simulink model "power_13NodeTestFeeder_4VSC_PV_DEG_symmtrc_loads_"  (R2024b)
settings: Solver=ode15s  StartTime=0.0  StopTime=5  FixedStep=1e-6  MaxStep=1e-4  RelTol=1e-6  AbsTol=1e-8  EnableMultiTasking=on
PreLoadFcn:
  | %power_13NodeTestFeeder_init;
values from neighbouring files (symbols this model uses):
  a = 1.3    [init_para_with_symmtrc_loads.m]
  Cdc = 278e-3    (= 0.278)    [init_para_with_symmtrc_loads.m]
  fg = 60    [a01_scan_VSC_13_feeder.m]    (also in init_para_with_symmtrc_loads.m)
  Gn = 1000    [init_para_with_symmtrc_loads.m]
  H = 8    [init_para_with_symmtrc_loads.m]
  Ipv_n = Isc_n*(Rp+Rs)/Rp    (= 8.21426513558)    [init_para_with_symmtrc_loads.m]
  Isc_n = 8.21    [init_para_with_symmtrc_loads.m]
  k = 1.3806503e-23    [init_para_with_symmtrc_loads.m]    (also in ypm_plot_compare_ana_meas.m = 2)
  Kdroop = Sn/(Rdroop*60)    (= 4166666.66667)    [init_para_with_symmtrc_loads.m]
  KI = 0.0032    [init_para_with_symmtrc_loads.m]
  Ki_C = Rc/tau_C    (= 0.768)    [init_para_with_symmtrc_loads.m]
  Ki_DC = omega_DC^2*Cdc    [init_para_with_symmtrc_loads.m]
  ki_dvpp = kp_dvpp/Ti_dvpp    [init_para_with_symmtrc_loads.m]
  Ki_P = 1/(Ki_pq*tau_P)    [init_para_with_symmtrc_loads.m]
  Ki_PLL = Kp_PLL/tau_PLL    [init_para_with_symmtrc_loads.m]
  Kp_C = Lc/tau_C    (= 0.020372)    [init_para_with_symmtrc_loads.m]
  Kp_DC = 2*xi_DC*omega_DC*Cdc    [init_para_with_symmtrc_loads.m]
  kp_dvpp = -(2*Kdcgain)^-1    [init_para_with_symmtrc_loads.m]
  Kp_P = tau_C/(Ki_pq*tau_P)    [init_para_with_symmtrc_loads.m]
  Kp_PLL = xi_PLL*2*omega_PLL/Vp    [init_para_with_symmtrc_loads.m]
  KV = -0.123    [init_para_with_symmtrc_loads.m]
  kv_Vp = [ 1.021 1.042 1.0174]    [init_para_with_symmtrc_loads.m]
  KVmp = Vmp_n/Voc_n    (= 0.799392097264)    [init_para_with_symmtrc_loads.m]
  Lc = 20.372e-6    (= 2.0372e-05)    [init_para_with_symmtrc_loads.m]
  Lg = Xg /(2*pi*fg)    [init_para_with_symmtrc_loads.m]
  Np = 345    [init_para_with_symmtrc_loads.m]
  Ns = 45    [init_para_with_symmtrc_loads.m]
  Ns_cell = 54    [init_para_with_symmtrc_loads.m]
  p_jump_time = 5    [init_para_with_symmtrc_loads.m]
  p_jump_value = 2*-1e6    (= -2000000)    [init_para_with_symmtrc_loads.m]
  phi_vec = phi_vec_deg/180*pi    [init_para_with_symmtrc_loads.m]
  ppv_nom = 4.9687e+05    (= 496870)    [init_para_with_symmtrc_loads.m]
  q = 1.6021764e-19    [init_para_with_symmtrc_loads.m]
  Rc = 0.768e-3    (= 0.000768)    [init_para_with_symmtrc_loads.m]
  Rg = (U_rms^2 / S_sc) / (sqrt(1 + XoverR^2))    [init_para_with_symmtrc_loads.m]
  Rp = 425.405    [init_para_with_symmtrc_loads.m]
  Rs = 0.221    [init_para_with_symmtrc_loads.m]
  S_base_all = 1    [init_para_with_symmtrc_loads.m]
  Sn = 15e6    (= 15000000)    [init_para_with_symmtrc_loads.m]
  tau_PLL = 2*xi_PLL/omega_PLL    [init_para_with_symmtrc_loads.m]
  Tn = 25    [init_para_with_symmtrc_loads.m]
  Ts = T_ctrl/n_ctrl    [a01_scan_VSC_13_feeder.m]    (also in init_para_with_symmtrc_loads.m = 5e-05)
  U_rms = 4160    [init_para_with_symmtrc_loads.m]
  Vdc = 1200    [init_para_with_symmtrc_loads.m]
  Voc_n = 32.9    [init_para_with_symmtrc_loads.m]
  Vp = sqrt(2)*480/sqrt(3)    [a01_scan_VSC_13_feeder.m]    (also in init_para_with_symmtrc_loads.m = Ug*sqrt(2)/sqrt(3))
undefined symbols (not defined in the file or in its folder): j, Newton, para_grid, para_PVgeno, Raphson
libraries: spsabctoAlphaBetaZeroLib x141, spsPower3phInstantaneousLib x70, spsSeriesRLCBranchLib x44, spsThreePhaseVIMeasurementLib x27, slpidlib x24, spsThreePhaseSeriesRLCLoadLib x15, spsControlledVoltageSourceLib x15, spsMeanLib x9, spsCurrentMeasurementLib x8, spsControlledCurrentSourceLib x8, cstblocks x8, spsGroundLib x5
(part 1 of 10)
settings Model: Creator=MathWorks  LastModifiedBy=clubbert
settings DataIOCC: ExternalInput=getinputstruct(op_IEEE_13_node_5)  InitialState=getstatestruct(op_IEEE_13_node_5)  LimitDataPoints=on  SaveFormat=Array  SignalLoggingSaveFormat=ModelDataLogs  ReturnWorkspaceOutputs=off
settings OptimizationCC: ExpressionDepthLimit=2147483647  LifeSpan=inf
settings DebuggingCC: UnderspecifiedInitializationDetection=Classic  MergeDetectMultiDrivingBlocksExec=none  FcnCallInpInsideContextMsg=warning  AllowSymbolicDim=off  StateNameClashWarn=warning  SFUnexpectedBacktrackingDiag=warning  SFNoUnconditionalDefaultTransitionDiag=warning  SFExecutionAtInitializationDiag=none  ArithmeticOperatorsInVariantConditions=warning
settings HardwareCC: ProdBitPerPointer=32  ProdBitPerSizeT=32  ProdBitPerPtrDiffT=32  ProdLargestAtomicFloat=None  ProdIntDivRoundTo=Undefined  ProdEndianess=Unspecified  ProdWordSize=32  ProdHWDeviceType=32-bit Generic
settings ModelReferenceCC: EnableRefExpFcnMdlSchedulingChecks=on  PropagateSignalLabelsOutOfModel=off
settings SFSimCC: SimUseLocalCustomCode=off  CustomCodeUndefinedFunction=UseInterfaceOnly
settings RTWCC: RTWUseLocalCustomCode=off  GPUComputeCapability=3.5
settings CodeAppCC: StateflowObjectComments=on
settings GRTTargetCC: TargetLangStandard=C89/C90 (ANSI)  CombineOutputUpdateFcns=off  GRTInterface=on
settings ConfigComp: CovMetricSettings=dw  CovSaveCumulativeToWorkspaceVar=on  CovSaveSingleToWorkspaceVar=on  CovExternalEMLEnable=off  CovSFcnEnable=off
settings SimscapeCC: SimscapeNormalizeSystem=off

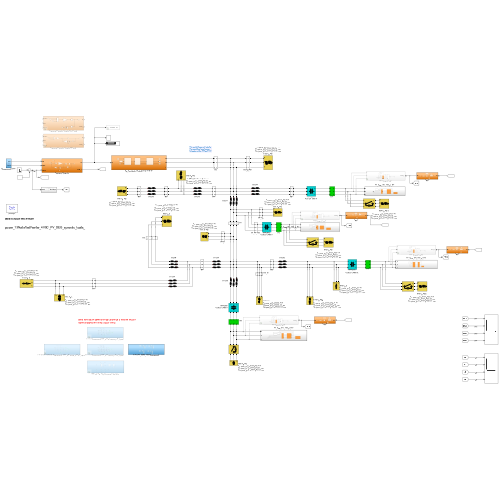
[thumbnail: Simulink's stored preview of the top-level diagram]
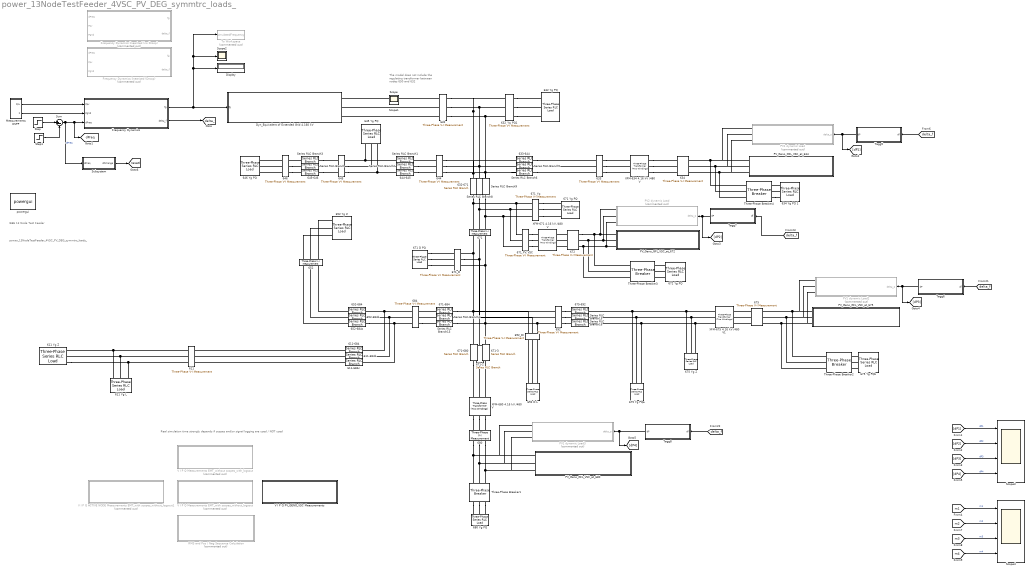
== system power_13NodeTestFeeder_4VSC_PV_DEG_symmtrc_loads_ ==
  note: Real simulation time strongly depends if scopes and/or
      | signal logging are used / NOT used
  note: power_13NodeTestFeeder_4VSC_PV_DEG_symmtrc_loads_
  note: IEEE 13 Node Test Feeder
  note: The model does not include
      | the regulating transformer
      | between nodes 650 and 632
  " 634 Yg PQ 1" : spsThreePhaseSeriesRLCLoadLib/Three-Phase Series RLC Load  LConnTagsString=A|B|C  Configuration=Y (grounded)  NominalVoltage=120e3  Vabc=para_grid.n634YgPQ.V_LN_rms  Vabcp=[1e3 1e3 1e3]  NominalFrequency=fg  UnbalancedPower=on  ActivePower=1e+006  InductivePower=0  CapacitivePower=0  Pabc=para_grid.n634YgPQ.P  QLabc=para_grid.n634YgPQ.QL  QCabc=para_grid.n634YgPQ.QC  Pabcp=[10e3 9e3 11e3]  QLabcp=[100 90 110]  QCabcp=[100 90 110]  Measurements=None  LoadType=constant PQ
      settings: AttributesFormatString=|
      | P= %<Pabc> W
      | Ql=%<QLabc> var
      | Qc=%<QCabc> var
  " 645 Yg PQ" : spsThreePhaseSeriesRLCLoadLib/Three-Phase Series RLC Load  LConnTagsString=A|B|C  Configuration=Y (grounded)  NominalVoltage=120e3  Vabc=para_grid.n645YgPQ.V_LN_rms  Vabcp=[1e3 1e3 1e3]  NominalFrequency=fg  UnbalancedPower=on  ActivePower=1e+006  InductivePower=0  CapacitivePower=0  Pabc=para_grid.n645YgPQ.P  QLabc=para_grid.n645YgPQ.QL  QCabc=para_grid.n645YgPQ.QC  Pabcp=[10e3 9e3 11e3]  QLabcp=[100 90 110]  QCabcp=[100 90 110]  Measurements=None  LoadType=constant PQ
      settings: AttributesFormatString=|
      | P= %<Pabc> W
      | Ql=%<QLabc> var
      | Qc=%<QCabc> var
  " 646 Yg PQ" : spsThreePhaseSeriesRLCLoadLib/Three-Phase Series RLC Load  LConnTagsString=A|B|C  Configuration=Y (grounded)  NominalVoltage=120e3  Vabc=para_grid.n646YgPQ.V_LN_rms  Vabcp=[1e3 1e3 1e3]  NominalFrequency=fg  UnbalancedPower=on  ActivePower=1e+006  InductivePower=0  CapacitivePower=0  Pabc=para_grid.n646YgPQ.P  QLabc=para_grid.n646YgPQ.QL  QCabc=para_grid.n646YgPQ.QC  Pabcp=[10e3 9e3 11e3]  QLabcp=[100 90 110]  QCabcp=[100 90 110]  Measurements=None  LoadType=constant PQ
      settings: AttributesFormatString=|
      | P= %<Pabc> W
      | Ql=%<QLabc> var
      | Qc=%<QCabc> var
  " 652 Yg Z" : spsThreePhaseSeriesRLCLoadLib/Three-Phase Series RLC Load  LConnTagsString=A|B|C  Configuration=Y (grounded)  NominalVoltage=120e3  Vabc=para_grid.n652YgZ.V_LN_rms  Vabcp=[1e3 1e3 1e3]  NominalFrequency=fg  UnbalancedPower=on  ActivePower=1e+006  InductivePower=0  CapacitivePower=0  Pabc=para_grid.n652YgZ.P  QLabc=para_grid.n652YgZ.QL  QCabc=para_grid.n652YgZ.QC  Pabcp=[10e3 9e3 11e3]  QLabcp=[100 90 110]  QCabcp=[100 90 110]  Measurements=None  LoadType=constant PQ
      settings: AttributesFormatString=|
      | P= %<Pabc> W
      | Ql=%<QLabc> var
      | Qc=%<QCabc> var
  " 672 Yg PQ " : spsThreePhaseSeriesRLCLoadLib/Three-Phase Series RLC Load  LConnTagsString=A|B|C  Configuration=Y (grounded)  NominalVoltage=120e3  Vabc=para_grid.n672YgPQ.V_LN_rms  Vabcp=[1e3 1e3 1e3]  NominalFrequency=fg  UnbalancedPower=on  ActivePower=1e+006  InductivePower=0  CapacitivePower=0  Pabc=para_grid.n672YgPQ.P  QLabc=para_grid.n672YgPQ.QL  QCabc=para_grid.n672YgPQ.QC  Pabcp=[10e3 9e3 11e3]  QLabcp=[100 90 110]  QCabcp=[100 90 110]  Measurements=None  LoadType=constant PQ
      settings: AttributesFormatString=|
      | P= %<Pabc> W
      | Ql=%<QLabc> var
      | Qc=%<QCabc> var
  " 675 Yg PQb " : spsThreePhaseSeriesRLCLoadLib/Three-Phase Series RLC Load  LConnTagsString=A|B|C  Configuration=Y (grounded)  NominalVoltage=120e3  Vabc=[ 0.993805 1.0218 0.995862]*277.128  Vabcp=[1e3 1e3 1e3]  NominalFrequency=60  UnbalancedPower=on  ActivePower=1e+006  InductivePower=0  CapacitivePower=0  Pabc=para_grid.n675YgPQb.P  QLabc=para_grid.n675YgPQb.QL  QCabc=para_grid.n675YgPQb.QC  Pabcp=[10e3 9e3 11e3]  QLabcp=[100 90 110]  QCabcp=[100 90 110]  Measurements=None  LoadType=constant PQ
      settings: AttributesFormatString=|
      | P= %<Pabc> W
      | Ql=%<QLabc> var
      | Qc=%<QCabc> var
  " 680 Yg PQ " : spsThreePhaseSeriesRLCLoadLib/Three-Phase Series RLC Load  LConnTagsString=A|B|C  Configuration=Y (grounded)  NominalVoltage=120e3  Vabc=para_grid.n680YgPQ.V_LN_rms  Vabcp=[1e3 1e3 1e3]  NominalFrequency=fg  UnbalancedPower=on  ActivePower=1e+006  InductivePower=0  CapacitivePower=0  Pabc=para_grid.n680YgPQ.P  QLabc=para_grid.n680YgPQ.QL  QCabc=para_grid.n680YgPQ.QC  Pabcp=[10e3 9e3 11e3]  QLabcp=[100 90 110]  QCabcp=[100 90 110]  Measurements=None  LoadType=constant PQ
      settings: AttributesFormatString=|
      | P= %<Pabc> W
      | Ql=%<QLabc> var
      | Qc=%<QCabc> var
  611 : spsThreePhaseVIMeasurementLib/Three-Phase V-I Measurement  VoltageMeasurement=phase-to-ground  SetLabelV=on  LabelV=Vabc_611  Vpu=off  VpuLL=off  CurrentMeasurement=yes  SetLabelI=on  LabelI=Iabc_611  Ipu=off  Pbase=100e6  Vbase=4160  OutputType=Complex  PhasorSimulation=off  PSBequivalent=0
  611 Yg L : spsThreePhaseSeriesRLCLoadLib/Three-Phase Series RLC Load  LConnTagsString=A|B|C  Configuration=Y (grounded)  NominalVoltage=120e3  Vabc=para_grid.n611YgL.V_LN_rms  Vabcp=para_grid.n671DPQ.V_LN_rms  NominalFrequency=fg  UnbalancedPower=on  ActivePower=1e+006  InductivePower=0  CapacitivePower=0  Pabc=para_grid.n611YgL.P  QLabc=para_grid.n611YgL.QL  QCabc=para_grid.n611YgL.QC  Pabcp=para_grid.n671DPQ.P  QLabcp=para_grid.n671DPQ.QL  QCabcp=para_grid.n671DPQ.QC  Measurements=None  LoadType=constant PQ
      settings: AttributesFormatString=|
      | P= %<Pabcp> W
      | Ql=%<QLabcp> var
      | Qc=%<QCabcp> var
  611 Yg Z : spsThreePhaseSeriesRLCLoadLib/Three-Phase Series RLC Load  LConnTagsString=A|B|C  Configuration=Y (grounded)  NominalVoltage=120e3  Vabc=para_grid.n611YgZ.V_LN_rms  Vabcp=para_grid.n671DPQ.V_LN_rms  NominalFrequency=fg  UnbalancedPower=on  ActivePower=1e+006  InductivePower=0  CapacitivePower=0  Pabc=para_grid.n611YgZ.P  QLabc=para_grid.n611YgZ.QL  QCabc=para_grid.n611YgZ.QC  Pabcp=para_grid.n671DPQ.P  QLabcp=para_grid.n671DPQ.QL  QCabcp=para_grid.n671DPQ.QC  Measurements=None  LoadType=constant PQ
      settings: AttributesFormatString=|
      | P= %<Pabcp> W
      | Ql=%<QLabcp> var
      | Qc=%<QCabcp> var
  611-684 : spsSeriesRLCBranchLib/Series RLC Branch  LConnTagsString=__new0  RConnTagsString=__new0  BranchType=RL  Resistance=para_grid.l611_684.R  Inductance=para_grid.l611_684.L  SetiL0=off  InitialCurrent=0  Capacitance=1e-6  Setx0=off  InitialVoltage=0  Measurements=None
  611-684b : spsSeriesRLCBranchLib/Series RLC Branch  LConnTagsString=__new0  RConnTagsString=__new0  BranchType=RL  Resistance=para_grid.l611_684.R  Inductance=para_grid.l611_684.L  SetiL0=off  InitialCurrent=0  Capacitance=1e-6  Setx0=off  InitialVoltage=0  Measurements=None
  611-684c : spsSeriesRLCBranchLib/Series RLC Branch  LConnTagsString=__new0  RConnTagsString=__new0  BranchType=RL  Resistance=para_grid.l611_684.R  Inductance=para_grid.l611_684.L  SetiL0=off  InitialCurrent=0  Capacitance=1e-6  Setx0=off  InitialVoltage=0  Measurements=None
  632 : spsThreePhaseVIMeasurementLib/Three-Phase V-I Measurement  VoltageMeasurement=phase-to-ground  SetLabelV=on  LabelV=Vabc_632  Vpu=off  VpuLL=off  CurrentMeasurement=yes  SetLabelI=on  LabelI=Iabc_632  Ipu=off  Pbase=100e6  Vbase=4160  OutputType=Complex  PhasorSimulation=off  PSBequivalent=0
  632 Yg PQ : spsThreePhaseSeriesRLCLoadLib/Three-Phase Series RLC Load  LConnTagsString=A|B|C  Configuration=Y (grounded)  NominalVoltage=120e3  Vabc=para_grid.n632YgPQ.V_LN_rms  Vabcp=[1e3 1e3 1e3]  NominalFrequency=fg  UnbalancedPower=on  ActivePower=1e+006  InductivePower=0  CapacitivePower=0  Pabc=para_grid.n632YgPQ.P  QLabc=para_grid.n632YgPQ.QL  QCabc=para_grid.n632YgPQ.QC  Pabcp=[10e3 9e3 11e3]  QLabcp=[100 90 110]  QCabcp=[100 90 110]  Measurements=None  LoadType=constant PQ
      settings: AttributesFormatString=|
      | P= %<Pabc> W
      | Ql=%<QLabc> var
      | Qc=%<QCabc> var
  632-671 : spsSeriesRLCBranchLib/Series RLC Branch  LConnTagsString=__new0  RConnTagsString=__new0  BranchType=RL  Resistance=para_grid.l632_671.R  Inductance=para_grid.l632_671.L  SetiL0=off  InitialCurrent=0  Capacitance=1e-6  Setx0=off  InitialVoltage=0  Measurements=None
  632_Yg_PQ1 : spsThreePhaseVIMeasurementLib/Three-Phase V-I Measurement  VoltageMeasurement=phase-to-ground  SetLabelV=on  LabelV=Vabc_632_Yg  Vpu=off  VpuLL=off  CurrentMeasurement=yes  SetLabelI=on  LabelI=Iabc_632_Yg  Ipu=off  Pbase=100e6  Vbase=4160  OutputType=Complex  PhasorSimulation=off  PSBequivalent=0
  633 : spsThreePhaseVIMeasurementLib/Three-Phase V-I Measurement  VoltageMeasurement=phase-to-ground  SetLabelV=on  LabelV=Vabc_633  Vpu=off  VpuLL=off  CurrentMeasurement=yes  SetLabelI=on  LabelI=Iabc_633  Ipu=off  Pbase=100e6  Vbase=4160  OutputType=Complex  PhasorSimulation=off  PSBequivalent=0
  633-644 : spsSeriesRLCBranchLib/Series RLC Branch  LConnTagsString=__new0  RConnTagsString=__new0  BranchType=RL  Resistance=para_grid.l633_644.R  Inductance=para_grid.l633_644.L  SetiL0=off  InitialCurrent=0  Capacitance=1e-6  Setx0=off  InitialVoltage=0  Measurements=None
  634 : spsThreePhaseVIMeasurementLib/Three-Phase V-I Measurement  VoltageMeasurement=phase-to-ground  SetLabelV=on  LabelV=Vabc_634  Vpu=off  VpuLL=off  CurrentMeasurement=yes  SetLabelI=on  LabelI=Iabc_634  Ipu=off  Pbase=100e6  Vbase=4160  OutputType=Complex  PhasorSimulation=off  PSBequivalent=0
  644 : spsThreePhaseVIMeasurementLib/Three-Phase V-I Measurement  VoltageMeasurement=phase-to-ground  SetLabelV=on  LabelV=Vabc_644  Vpu=off  VpuLL=off  CurrentMeasurement=yes  SetLabelI=on  LabelI=Iabc_644  Ipu=off  Pbase=100e6  Vbase=4160  OutputType=Complex  PhasorSimulation=off  PSBequivalent=0
  644-645 : spsSeriesRLCBranchLib/Series RLC Branch  LConnTagsString=__new0  RConnTagsString=__new0  BranchType=RL  Resistance=para_grid.l644_645.R  Inductance=para_grid.l644_645.L  SetiL0=off  InitialCurrent=0  Capacitance=1e-6  Setx0=off  InitialVoltage=0  Measurements=None
  645 : spsThreePhaseVIMeasurementLib/Three-Phase V-I Measurement  VoltageMeasurement=phase-to-ground  SetLabelV=on  LabelV=Vabc_645  Vpu=off  VpuLL=off  CurrentMeasurement=yes  SetLabelI=on  LabelI=Iabc_645  Ipu=off  Pbase=100e6  Vbase=4160  OutputType=Complex  PhasorSimulation=off  PSBequivalent=0
  645-646 : spsSeriesRLCBranchLib/Series RLC Branch  LConnTagsString=__new0  RConnTagsString=__new0  BranchType=RL  Resistance=para_grid.l645_646.R  Inductance=para_grid.l645_646.L  SetiL0=off  InitialCurrent=0  Capacitance=1e-6  Setx0=off  InitialVoltage=0  Measurements=None
  646 : spsThreePhaseVIMeasurementLib/Three-Phase V-I Measurement  VoltageMeasurement=phase-to-ground  SetLabelV=on  LabelV=Vabc_646  Vpu=off  VpuLL=off  CurrentMeasurement=yes  SetLabelI=on  LabelI=Iabc_646  Ipu=off  Pbase=100e6  Vbase=4160  OutputType=Complex  PhasorSimulation=off  PSBequivalent=0
  652 : spsThreePhaseVIMeasurementLib/Three-Phase V-I Measurement  VoltageMeasurement=phase-to-ground  SetLabelV=on  LabelV=Vabc_652  Vpu=off  VpuLL=off  CurrentMeasurement=yes  SetLabelI=on  LabelI=Iabc_652  Ipu=off  Pbase=100e6  Vbase=4160  OutputType=Complex  PhasorSimulation=off  PSBequivalent=0
  652-684 : spsSeriesRLCBranchLib/Series RLC Branch  LConnTagsString=__new0  RConnTagsString=__new0  BranchType=RL  Resistance=para_grid.l652_684.R  Inductance=para_grid.l652_684.L  SetiL0=off  InitialCurrent=0  Capacitance=1e-6  Setx0=off  InitialVoltage=0  Measurements=None
  652-684b : spsSeriesRLCBranchLib/Series RLC Branch  LConnTagsString=__new0  RConnTagsString=__new0  BranchType=RL  Resistance=para_grid.l652_684.R  Inductance=para_grid.l652_684.L  SetiL0=off  InitialCurrent=0  Capacitance=1e-6  Setx0=off  InitialVoltage=0  Measurements=None
  652-684c : spsSeriesRLCBranchLib/Series RLC Branch  LConnTagsString=__new0  RConnTagsString=__new0  BranchType=RL  Resistance=para_grid.l652_684.R  Inductance=para_grid.l652_684.L  SetiL0=off  InitialCurrent=0  Capacitance=1e-6  Setx0=off  InitialVoltage=0  Measurements=None
  671 : spsThreePhaseVIMeasurementLib/Three-Phase V-I Measurement  VoltageMeasurement=phase-to-ground  SetLabelV=on  LabelV=Vabc_671  Vpu=off  VpuLL=off  CurrentMeasurement=yes  SetLabelI=on  LabelI=Iabc_671  Ipu=off  Pbase=100e6  Vbase=4160  OutputType=Complex  PhasorSimulation=off  PSBequivalent=0
  671 D PQ : spsThreePhaseSeriesRLCLoadLib/Three-Phase Series RLC Load  LConnTagsString=A|B|C  Configuration=Delta  NominalVoltage=120e3  Vabc="[1  1  1]*120e3/sqrt(3)"  Vabcp=para_grid.n671DPQ.V_LN_rms  NominalFrequency=fg  UnbalancedPower=on  ActivePower=1e+006  InductivePower=0  CapacitivePower=0  Pabc="[17 66  117]*1e3/2"  QLabc="[10 38  68]*1e3/2"  QCabc=[0 0 0]  Pabcp=para_grid.n671DPQ.P  QLabcp=para_grid.n671DPQ.QL  QCabcp=para_grid.n671DPQ.QC  Measurements=None  LoadType=constant PQ
      settings: AttributesFormatString=|
      | P= %<Pabcp> W
      | Ql=%<QLabcp> var
      | Qc=%<QCabcp> var
  671 Yg PQ : spsThreePhaseSeriesRLCLoadLib/Three-Phase Series RLC Load  LConnTagsString=A|B|C  Configuration=Y (grounded)  NominalVoltage=120e3  Vabc=para_grid.n671YgPQ.V_LN_rms  Vabcp=[1e3 1e3 1e3]  NominalFrequency=fg  UnbalancedPower=on  ActivePower=1e+006  InductivePower=0  CapacitivePower=0  Pabc=para_grid.n671YgPQ.P  QLabc=para_grid.n671YgPQ.QL  QCabc=para_grid.n671YgPQ.QC  Pabcp=[10e3 9e3 11e3]  QLabcp=[100 90 110]  QCabcp=[100 90 110]  Measurements=None  LoadType=constant PQ
      settings: AttributesFormatString=|
      | P= %<Pabc> W
      | Ql=%<QLabc> var
      | Qc=%<QCabc> var
  671-2 : spsSeriesRLCBranchLib/Series RLC Branch  LConnTagsString=__new0  RConnTagsString=__new0  BranchType=RL  Resistance=para_grid.l671_680.R  Inductance=para_grid.l671_680.L  SetiL0=off  InitialCurrent=0  Capacitance=1e-6  Setx0=off  InitialVoltage=0  Measurements=None
  671-3 : spsSeriesRLCBranchLib/Series RLC Branch  LConnTagsString=__new0  RConnTagsString=__new0  BranchType=RL  Resistance=para_grid.l671_680.R  Inductance=para_grid.l671_680.L  SetiL0=off  InitialCurrent=0  Capacitance=1e-6  Setx0=off  InitialVoltage=0  Measurements=None
  671-680 : spsSeriesRLCBranchLib/Series RLC Branch  LConnTagsString=__new0  RConnTagsString=__new0  BranchType=RL  Resistance=para_grid.l671_680.R  Inductance=para_grid.l671_680.L  SetiL0=off  InitialCurrent=0  Capacitance=1e-6  Setx0=off  InitialVoltage=0  Measurements=None
  671-684 : spsSeriesRLCBranchLib/Series RLC Branch  LConnTagsString=__new0  RConnTagsString=__new0  BranchType=RL  Resistance=para_grid.l671_684.R  Inductance=para_grid.l671_684.L  SetiL0=off  InitialCurrent=0  Capacitance=1e-6  Setx0=off  InitialVoltage=0  Measurements=None
  671_D : spsThreePhaseVIMeasurementLib/Three-Phase V-I Measurement  VoltageMeasurement=phase-to-ground  SetLabelV=on  LabelV=Vabc_671_D  Vpu=off  VpuLL=off  CurrentMeasurement=yes  SetLabelI=on  LabelI=Iabc_671_D  Ipu=off  Pbase=100e6  Vbase=4160  OutputType=Complex  PhasorSimulation=off  PSBequivalent=0
  671_PV_VSC : spsThreePhaseVIMeasurementLib/Three-Phase V-I Measurement  VoltageMeasurement=phase-to-ground  SetLabelV=on  LabelV=Vabc_671_VSC  Vpu=off  VpuLL=off  CurrentMeasurement=yes  SetLabelI=on  LabelI=Iabc_671_VSC  Ipu=off  Pbase=100e6  Vbase=4160  OutputType=Complex  PhasorSimulation=off  PSBequivalent=0
  671_Yg : spsThreePhaseVIMeasurementLib/Three-Phase V-I Measurement  VoltageMeasurement=phase-to-ground  SetLabelV=on  LabelV=Vabc_671_Yg  Vpu=off  VpuLL=off  CurrentMeasurement=yes  SetLabelI=on  LabelI=Iabc_671_Yg  Ipu=off  Pbase=100e6  Vbase=4160  OutputType=Complex  PhasorSimulation=off  PSBequivalent=0
  672 : spsThreePhaseVIMeasurementLib/Three-Phase V-I Measurement  VoltageMeasurement=phase-to-ground  SetLabelV=on  LabelV=Vabc_672  Vpu=off  VpuLL=off  CurrentMeasurement=yes  SetLabelI=on  LabelI=Iabc_672  Ipu=off  Pbase=100e6  Vbase=4160  OutputType=Complex  PhasorSimulation=off  PSBequivalent=0
  675 : spsThreePhaseVIMeasurementLib/Three-Phase V-I Measurement  VoltageMeasurement=phase-to-ground  SetLabelV=on  LabelV=Vabc_675  Vpu=off  VpuLL=off  CurrentMeasurement=yes  SetLabelI=on  LabelI=Iabc_675  Ipu=off  Pbase=100e6  Vbase=4160  OutputType=Complex  PhasorSimulation=off  PSBequivalent=0
  675 Yg PQa : spsThreePhaseSeriesRLCLoadLib/Three-Phase Series RLC Load  LConnTagsString=A|B|C  Configuration=Y (grounded)  NominalVoltage=120e3  Vabc=para_grid.n675YgPQa.V_LN_rms  Vabcp=[1e3 1e3 1e3]  NominalFrequency=fg  UnbalancedPower=on  ActivePower=1e+006  InductivePower=0  CapacitivePower=0  Pabc=para_grid.n675YgPQa.P  QLabc=para_grid.n675YgPQa.QL  QCabc=para_grid.n675YgPQa.QC  Pabcp=[10e3 9e3 11e3]  QLabcp=[100 90 110]  QCabcp=[100 90 110]  Measurements=None  LoadType=constant PQ
      settings: AttributesFormatString=|
      | P= %<Pabc> W
      | Ql=%<QLabc> var
      | Qc=%<QCabc> var
  675 Yg Z : spsThreePhaseSeriesRLCLoadLib/Three-Phase Series RLC Load  LConnTagsString=A|B|C  Configuration=Y (grounded)  NominalVoltage=120e3  Vabc=para_grid.n675YgZ.V_LN_rms  Vabcp=[1e3 1e3 1e3]  NominalFrequency=fg  UnbalancedPower=on  ActivePower=1e+006  InductivePower=0  CapacitivePower=0  Pabc=para_grid.n675YgZ.P  QLabc=para_grid.n675YgZ.QL  QCabc=para_grid.n675YgZ.QC  Pabcp=[10e3 9e3 11e3]  QLabcp=[100 90 110]  QCabcp=[100 90 110]  Measurements=None  LoadType=constant Z
      settings: AttributesFormatString=|
      | P= %<Pabc> W
      | Ql=%<QLabc> var
      | Qc=%<QCabc> var
  675-692 : spsSeriesRLCBranchLib/Series RLC Branch  LConnTagsString=__new0  RConnTagsString=__new0  BranchType=RL  Resistance=para_grid.l675_692.R  Inductance=para_grid.l675_692.L  SetiL0=off  InitialCurrent=0  Capacitance=1e-6  Setx0=off  InitialVoltage=0  Measurements=None
  680 : spsThreePhaseVIMeasurementLib/Three-Phase V-I Measurement  VoltageMeasurement=phase-to-ground  SetLabelV=on  LabelV=Vabc_680  Vpu=off  VpuLL=off  CurrentMeasurement=yes  SetLabelI=on  LabelI=Iabc_680  Ipu=off  Pbase=100e6  Vbase=4160  OutputType=Complex  PhasorSimulation=off  PSBequivalent=0
  684 : spsThreePhaseVIMeasurementLib/Three-Phase V-I Measurement  VoltageMeasurement=phase-to-ground  SetLabelV=on  LabelV=Vabc_684  Vpu=off  VpuLL=off  CurrentMeasurement=yes  SetLabelI=on  LabelI=Iabc_684  Ipu=off  Pbase=100e6  Vbase=4160  OutputType=Complex  PhasorSimulation=off  PSBequivalent=0
  692 : spsThreePhaseVIMeasurementLib/Three-Phase V-I Measurement  VoltageMeasurement=phase-to-ground  SetLabelV=on  LabelV=Vabc_692  Vpu=off  VpuLL=off  CurrentMeasurement=yes  SetLabelI=on  LabelI=Iabc_692  Ipu=off  Pbase=100e6  Vbase=4160  OutputType=Complex  PhasorSimulation=off  PSBequivalent=0
  692 D L : spsThreePhaseSeriesRLCLoadLib/Three-Phase Series RLC Load  LConnTagsString=A|B|C  Configuration=Delta  NominalVoltage=120e3  Vabc="[1  1  1]*120e3/sqrt(3)"  Vabcp=para_grid.n692DL.V_LN_rms  NominalFrequency=fg  UnbalancedPower=on  ActivePower=1e+006  InductivePower=0  CapacitivePower=0  Pabc="[17 66  117]*1e3/2"  QLabc="[10 38  68]*1e3/2"  QCabc=[0 0 0]  Pabcp=para_grid.n692DL.P  QLabcp=para_grid.n692DL.QL  QCabcp=para_grid.n692DL.QC  Measurements=None  LoadType=constant I
      settings: AttributesFormatString=|
      | P= %<Pabcp> W
      | Ql=%<QLabcp> var
      | Qc=%<QCabcp> var
  692_DI : spsThreePhaseVIMeasurementLib/Three-Phase V-I Measurement  VoltageMeasurement=phase-to-ground  SetLabelV=on  LabelV=Vabc_692_DI  Vpu=off  VpuLL=off  CurrentMeasurement=yes  SetLabelI=on  LabelI=Iabc_692_DI  Ipu=off  Pbase=100e6  Vbase=4160  OutputType=Complex  PhasorSimulation=off  PSBequivalent=0
  Display : Display
  Dyn_Equivalent of Extended Grid 4.160 kV : Subsystem
  Frequency Dynamics : Subsystem
  Frequency Dynamics linearized (Droop) : Subsystem  Commented=on
  Frequency Dynamics linearized (no Droop) : Subsystem  Commented=on
  Measurements DVPP : Subsystem
  PV1 dynamic Load : Subsystem  Commented=on
  PV1 dynamic Load2 : Subsystem  Commented=on
  PV1 dynamic Load3 : Subsystem  Commented=on
  PV2 dynamic Load : Subsystem  Commented=on
  PV_Geno_GFL_VSC_at_634 : Subsystem
  PV_Geno_GFL_VSC_at_672 : Subsystem
  PV_Geno_GFL_VSC_at_675 : Subsystem
  PV_Geno_GFL_VSC_at_680 : Subsystem
  "RMS and Pos / Neg Sequence Calculation " : Subsystem  Commented=on
  Scope2 : Scope
  Scope3 : Scope  NumInputPorts=4
  Scope4 : Scope  NumInputPorts=4
  Series RLC Branch : spsSeriesRLCBranchLib/Series RLC Branch  LConnTagsString=__new0  RConnTagsString=__new0  BranchType=RL  Resistance=para_grid.l645_646.R  Inductance=para_grid.l645_646.L  SetiL0=off  InitialCurrent=0  Capacitance=1e-6  Setx0=off  InitialVoltage=0  Measurements=None
  Series RLC Branch1 : spsSeriesRLCBranchLib/Series RLC Branch  LConnTagsString=__new0  RConnTagsString=__new0  BranchType=RL  Resistance=para_grid.l644_645.R  Inductance=para_grid.l644_645.L  SetiL0=off  InitialCurrent=0  Capacitance=1e-6  Setx0=off  InitialVoltage=0  Measurements=None
  Series RLC Branch13 : spsSeriesRLCBranchLib/Series RLC Branch  LConnTagsString=__new0  RConnTagsString=__new0  BranchType=RL  Resistance=para_grid.l671_684.R  Inductance=para_grid.l671_684.L  SetiL0=off  InitialCurrent=0  Capacitance=1e-6  Setx0=off  InitialVoltage=0  Measurements=None
  Series RLC Branch15 : spsSeriesRLCBranchLib/Series RLC Branch  LConnTagsString=__new0  RConnTagsString=__new0  BranchType=RL  Resistance=para_grid.l675_692.R  Inductance=para_grid.l675_692.L  SetiL0=off  InitialCurrent=0  Capacitance=1e-6  Setx0=off  InitialVoltage=0  Measurements=None
  Series RLC Branch16 : spsSeriesRLCBranchLib/Series RLC Branch  LConnTagsString=__new0  RConnTagsString=__new0  BranchType=RL  Resistance=para_grid.l675_692.R  Inductance=para_grid.l675_692.L  SetiL0=off  InitialCurrent=0  Capacitance=1e-6  Setx0=off  InitialVoltage=0  Measurements=None
  Series RLC Branch2 : spsSeriesRLCBranchLib/Series RLC Branch  LConnTagsString=__new0  RConnTagsString=__new0  BranchType=RL  Resistance=para_grid.l644_645.R  Inductance=para_grid.l644_645.L  SetiL0=off  InitialCurrent=0  Capacitance=1e-6  Setx0=off  InitialVoltage=0  Measurements=None
  Series RLC Branch3 : spsSeriesRLCBranchLib/Series RLC Branch  LConnTagsString=__new0  RConnTagsString=__new0  BranchType=RL  Resistance=para_grid.l645_646.R  Inductance=para_grid.l645_646.L  SetiL0=off  InitialCurrent=0  Capacitance=1e-6  Setx0=off  InitialVoltage=0  Measurements=None
  Series RLC Branch4 : spsSeriesRLCBranchLib/Series RLC Branch  LConnTagsString=__new0  RConnTagsString=__new0  BranchType=RL  Resistance=para_grid.l671_684.R  Inductance=para_grid.l671_684.L  SetiL0=off  InitialCurrent=0  Capacitance=1e-6  Setx0=off  InitialVoltage=0  Measurements=None
  Series RLC Branch5 : spsSeriesRLCBranchLib/Series RLC Branch  LConnTagsString=__new0  RConnTagsString=__new0  BranchType=RL  Resistance=para_grid.l633_644.R  Inductance=para_grid.l633_644.L  SetiL0=off  InitialCurrent=0  Capacitance=1e-6  Setx0=off  InitialVoltage=0  Measurements=None
  Series RLC Branch6 : spsSeriesRLCBranchLib/Series RLC Branch  LConnTagsString=__new0  RConnTagsString=__new0  BranchType=RL  Resistance=para_grid.l633_644.R  Inductance=para_grid.l633_644.L  SetiL0=off  InitialCurrent=0  Capacitance=1e-6  Setx0=off  InitialVoltage=0  Measurements=None
  Series RLC Branch8 : spsSeriesRLCBranchLib/Series RLC Branch  LConnTagsString=__new0  RConnTagsString=__new0  BranchType=RL  Resistance=para_grid.l632_671.R  Inductance=para_grid.l632_671.L  SetiL0=off  InitialCurrent=0  Capacitance=1e-6  Setx0=off  InitialVoltage=0  Measurements=None
  Series RLC Branch9 : spsSeriesRLCBranchLib/Series RLC Branch  LConnTagsString=__new0  RConnTagsString=__new0  BranchType=RL  Resistance=para_grid.l632_671.R  Inductance=para_grid.l632_671.L  SetiL0=off  InitialCurrent=0  Capacitance=1e-6  Setx0=off  InitialVoltage=0  Measurements=None
  Step : Step  Time=p_jump_time  After=p_jump_value  SampleTime=0
  Step1 : Step  Time=p_jump_time+10  After=p_jump_value  SampleTime=0
  Subsystem : Subsystem
  Sum : Sum  Inputs=|+-
  Tagg5 : Subsystem
  Tagg6 : Subsystem
  Tagg7 : Subsystem
  Tagg8 : Subsystem
  Three-Phase Breaker1 : spsThreePhaseBreakerLib/Three-Phase Breaker  InitialState=open  SwitchA=on  SwitchB=on  SwitchC=on  SwitchTimes=para_grid.n680YgPQ.ts  External=off  BreakerResistance=0.01  SnubberResistance=1e6  SnubberCapacitance=inf  Measurements=None
  Three-Phase Breaker2 : spsThreePhaseBreakerLib/Three-Phase Breaker  InitialState=open  SwitchA=on  SwitchB=on  SwitchC=on  SwitchTimes=para_grid.n675YgPQ.ts  External=off  BreakerResistance=0.01  SnubberResistance=1e6  SnubberCapacitance=inf  Measurements=None
  Three-Phase Breaker3 : spsThreePhaseBreakerLib/Three-Phase Breaker  InitialState=open  SwitchA=on  SwitchB=on  SwitchC=on  SwitchTimes=para_grid.n672YgPQ.ts  External=off  BreakerResistance=0.01  SnubberResistance=1e6  SnubberCapacitance=inf  Measurements=None
  Three-Phase Breaker4 : spsThreePhaseBreakerLib/Three-Phase Breaker  InitialState=open  SwitchA=on  SwitchB=on  SwitchC=on  SwitchTimes=para_grid.n634YgPQ.ts  External=off  BreakerResistance=0.01  SnubberResistance=1e6  SnubberCapacitance=inf  Measurements=None
  To Workspace : ToWorkspace  Commented=on  VariableName=simulatedFrequency  SaveFormat=Timeseries  SampleTime=Ts
  V I P Q ACTIVE NODE Measurements EMT_with scopes_without_logsout1 : Subsystem  Commented=on
  V I P Q Measurements EMT_with scopes_without_logsout : Subsystem  Commented=on
  V I P Q Measurements EMT_without scopes_with_logsout : Subsystem  Commented=on
  V I P Q PV_GENO_VSC Measurements : Subsystem
  XFM-634 4.16 kV /480 V : spsThreePhaseTransformerTwoWindingsLib/Three-Phase Transformer (Two Windings)  Winding1Connection=Yg  Winding2Connection=Yg  CoreType=Three single-phase transformers  SetSaturation=off  Hysteresis=off  DataFile='hysteresis'  SetInitialFlux=off  Measurements=None  UNITS=pu  NominalPower=[ 500e3 , 60 ]  Winding1=[4160 0.011 0.02]  Winding2=[480 0 0]  Rm=500  Lm=500  L0=0.5  Saturation=[0 0;0.0024 1.2;1 1.52]  InitialFluxes=[0.8 -0.8 0.7]  BreakLoop=off  DiscreteSolver=Trapezoidal iterative  DataType=off  TransfoNumber=1
  XFM-671 4.16 kV /480 V : spsThreePhaseTransformerTwoWindingsLib/Three-Phase Transformer (Two Windings)  Winding1Connection=Yg  Winding2Connection=Yg  CoreType=Three single-phase transformers  SetSaturation=off  Hysteresis=off  DataFile='hysteresis'  SetInitialFlux=off  Measurements=None  UNITS=pu  NominalPower=[ 500e3 , 60 ]  Winding1=[4160 0.011 0.02]  Winding2=[480 0 0]  Rm=500  Lm=500  L0=0.5  Saturation=[0 0;0.0024 1.2;1 1.52]  InitialFluxes=[0.8 -0.8 0.7]  BreakLoop=off  DiscreteSolver=Trapezoidal iterative  DataType=off  TransfoNumber=1
  XFM-675 4.16 kV /480 V1 : spsThreePhaseTransformerTwoWindingsLib/Three-Phase Transformer (Two Windings)  Winding1Connection=Yg  Winding2Connection=Yg  CoreType=Three single-phase transformers  SetSaturation=off  Hysteresis=off  DataFile='hysteresis'  SetInitialFlux=off  Measurements=None  UNITS=pu  NominalPower=[ 500e3 , 60 ]  Winding1=[4160 0.011 0.02]  Winding2=[480 0 0]  Rm=500  Lm=500  L0=0.5  Saturation=[0 0;0.0024 1.2;1 1.52]  InitialFluxes=[0.8 -0.8 0.7]  BreakLoop=off  DiscreteSolver=Trapezoidal iterative  DataType=off  TransfoNumber=1
  XFM-680 4.16 kV /480 V : spsThreePhaseTransformerTwoWindingsLib/Three-Phase Transformer (Two Windings)  Winding1Connection=Yg  Winding2Connection=Yg  CoreType=Three single-phase transformers  SetSaturation=off  Hysteresis=off  DataFile='hysteresis'  SetInitialFlux=off  Measurements=None  UNITS=pu  NominalPower=[ 500e3 , 60 ]  Winding1=[4160 0.011 0.02]  Winding2=[480 0 0]  Rm=500  Lm=500  L0=0.5  Saturation=[0 0;0.0024 1.2;1 1.52]  InitialFluxes=[0.8 -0.8 0.7]  BreakLoop=off  DiscreteSolver=Trapezoidal iterative  DataType=off  TransfoNumber=1
  powergui : spspowerguiLib/powergui  Priority=1  SimulationMode=Discrete  SampleTime=Ts  frequency=60  Iterations=50  frequencyindice=0  Pbase=100e3  ErrMax=0.0001  UnitsV=kV  UnitsW=kW  buscounter=0  FunctionMessages=off  echomessages=off  EnableUseOfTLC=off  CurrentSourceSwitches=off  DisableSnubberDevices=off  DisableRonSwitches=off  DisableVfSwitches=off  DisplayEquations=off  AutomaticDiscreteSolvers=off  SolverType=Tustin/Backward Euler (TBE)  Interpol=off  ExternalGateDelay=off  methode=off  Ts=0  x0status=blocks  SPID=off  SwTol=0  HookPort=off  NonlinearTolerance=1e-4  nMaxIteration=100  ContinueOnMaxIteration=off  RestoreLinks=warning  ResistiveCurrentMeasurement=off  Frange=[0:2:500]  Ylog=off  Xlog=on  ShowGrid=off  save=off  variable=ZData  structure=0  ZoomFFT=on  StartTime=0.0  cycles=1  DisplayStyle=1  fundamental=60  FreqAxis=off  MaxFrequency=1000  frequencyindicesteady=1  RmsSteady=1  display=off
  Scope : Scope
  Scope1 : Scope
  tag scope: dPreq=global, delta_f=global, resetI=global
  wires:
  Frequency Dynamics/2(delta_f) -> [delta_f]
  Frequency Dynamics/1(fg) -> Display/1, To Workspace/1, Scope2/1, Dyn_Equivalent of Extended Grid 4.160 kV/1(fg)
  Step/1 -> Sum/1
  Step1/1 -> Sum/2
  Measurements DVPP/2(Pgrid) -> Frequency Dynamics/2(Pgrid)
  Measurements DVPP/1(Ppv) -> Frequency Dynamics/1(Ppv)
  Sum/1 -> Subsystem/1(dPreq), [dPreq], Frequency Dynamics/3(dPreq)  "dPreq"
  [dP1] -> Scope3/1  "dP1"
  [dP2] -> Scope3/2  "dP2"
  [dP3] -> Scope3/3  "dP3"
  [dP4] -> Scope3/4  "dP4"
  Tagg5/1(dP) -> PV1 dynamic Load/1(delta_p), [dP1]
  Tagg7/1(dP) -> [dP2], PV2 dynamic Load/1(delta_p)
  Tagg6/1(dP) -> [dP3], PV1 dynamic Load2/1(delta_p)
  [delta_f] -> Tagg5/1(df)
  [delta_f] -> Tagg6/1(df)
  [delta_f] -> Tagg7/1(df)
  Tagg8/1(dP) -> [dP4], PV1 dynamic Load3/1(delta_p)
  [delta_f] -> Tagg8/1(df)
  Subsystem/1(dPchange) -> [resetI]
  [m4] -> Scope4/4  "m4"
  [m2] -> Scope4/2  "m2"
  [m1] -> Scope4/1  "m1"
  [m3] -> Scope4/3  "m3"
  connections:
  Series RLC Branch6/LConn1 -- Series RLC Branch9/LConn1 -- 644/LConn3 -- 632_Yg_PQ1/LConn3 -- 632/RConn3
  675 Yg PQa/LConn2 -- Series RLC Branch15/RConn1 -- 675 Yg Z/LConn2 -- XFM-675 4.16 kV /480 V1/LConn2
  675 Yg PQa/LConn3 -- Series RLC Branch16/RConn1 -- 675 Yg Z/LConn3 -- XFM-675 4.16 kV /480 V1/LConn3
  675 Yg PQa/LConn1 -- 675 Yg Z/LConn1 -- XFM-675 4.16 kV /480 V1/LConn1 -- 675-692/RConn1
  645/LConn2 -- Series RLC Branch2/LConn1 -- " 645 Yg PQ"/LConn2
  671-680/LConn1 -- 671-684/RConn1 -- 692/RConn1 -- 692_DI/LConn1 -- 671_D/LConn1 -- 671/RConn1
  611 Yg Z/LConn3 -- 611/RConn3 -- 611 Yg L/LConn3
  671_D/LConn2 -- 692_DI/LConn2 -- 692/RConn2 -- 671-2/LConn1 -- Series RLC Branch4/RConn1 -- 671/RConn2
  Series RLC Branch9/RConn1 -- 671/LConn3 -- 671_PV_VSC/RConn3 -- 671_Yg/RConn3
  632-671/LConn1 -- 632_Yg_PQ1/LConn1 -- 632/RConn1 -- 644/LConn1 -- 633-644/LConn1
  Series RLC Branch8/LConn1 -- 644/LConn2 -- Series RLC Branch5/LConn1 -- 632_Yg_PQ1/LConn2 -- 632/RConn2
  671 D PQ/LConn1 -- 671_D/RConn1
  671 D PQ/LConn2 -- 671_D/RConn2
  671 D PQ/LConn3 -- 671_D/RConn3
  671_Yg/LConn1 -- 671 Yg PQ/LConn1
  671_Yg/LConn2 -- 671 Yg PQ/LConn2
  671_Yg/LConn3 -- 671 Yg PQ/LConn3
  692 D L/LConn1 -- 692_DI/RConn1
  692 D L/LConn2 -- 692_DI/RConn2
  692 D L/LConn3 -- 692_DI/RConn3
  645/LConn3 -- 644-645/LConn1 -- " 645 Yg PQ"/LConn3
  Series RLC Branch/RConn1 -- 645/RConn2
  645-646/RConn1 -- 645/RConn3
  Series RLC Branch1/LConn1 -- 645/LConn1 -- " 645 Yg PQ"/LConn1
  Series RLC Branch3/LConn1 -- 646/LConn1
  646/RConn1 -- " 646 Yg PQ"/LConn1
  646/LConn2 -- Series RLC Branch/LConn1
  646/LConn3 -- 645-646/LConn1
  633-644/RConn1 -- 633/RConn1
  Series RLC Branch5/RConn1 -- 633/RConn2
  Series RLC Branch6/RConn1 -- 633/RConn3
  633/LConn1 -- XFM-634 4.16 kV /480 V/LConn1
  633/LConn2 -- XFM-634 4.16 kV /480 V/LConn2
  633/LConn3 -- XFM-634 4.16 kV /480 V/LConn3
  692_DI/LConn3 -- 692/RConn3 -- 671-3/LConn1 -- Series RLC Branch13/RConn1 -- 671/RConn3 -- 671_D/LConn3
  Series RLC Branch8/RConn1 -- 671/LConn2 -- 671_PV_VSC/RConn2 -- 671_Yg/RConn2
  632-671/RConn1 -- 671_PV_VSC/RConn1 -- 671_Yg/RConn1 -- 671/LConn1
  611-684c/LConn1 -- 611/LConn3
  652-684/RConn1 -- 652/LConn1
  692/LConn1 -- 675-692/LConn1
  692/LConn2 -- Series RLC Branch15/LConn1
  692/LConn3 -- Series RLC Branch16/LConn1
  644/RConn1 -- Series RLC Branch1/RConn1
  644-645/RConn1 -- 644/RConn3
  Series RLC Branch2/RConn1 -- 644/RConn2
  632_Yg_PQ1/RConn1 -- 632 Yg PQ/LConn1
  632_Yg_PQ1/RConn3 -- 632 Yg PQ/LConn3
  632_Yg_PQ1/RConn2 -- 632 Yg PQ/LConn2
  Three-Phase Breaker2/LConn1 -- PV1 dynamic Load2/RConn1 -- PV_Geno_GFL_VSC_at_675/RConn1 -- 675/LConn1
  Three-Phase Breaker2/LConn2 -- PV1 dynamic Load2/RConn2 -- PV_Geno_GFL_VSC_at_675/RConn2 -- 675/LConn2
  Three-Phase Breaker2/LConn3 -- PV1 dynamic Load2/RConn3 -- PV_Geno_GFL_VSC_at_675/RConn3 -- 675/LConn3
  " 675 Yg PQb "/LConn1 -- Three-Phase Breaker2/RConn1
  " 675 Yg PQb "/LConn2 -- Three-Phase Breaker2/RConn2
  " 675 Yg PQb "/LConn3 -- Three-Phase Breaker2/RConn3
  675/RConn1 -- XFM-675 4.16 kV /480 V1/RConn1
  675/RConn2 -- XFM-675 4.16 kV /480 V1/RConn2
  675/RConn3 -- XFM-675 4.16 kV /480 V1/RConn3
  684/RConn1 -- 611-684/RConn1 -- 652-684/LConn1
  671-684/LConn1 -- 684/LConn1
  684/RConn3 -- 652-684c/LConn1 -- 611-684c/RConn1
  684/LConn3 -- Series RLC Branch13/LConn1
  671_PV_VSC/LConn1 -- XFM-671 4.16 kV /480 V/LConn1
  671_PV_VSC/LConn2 -- XFM-671 4.16 kV /480 V/LConn2
  671_PV_VSC/LConn3 -- XFM-671 4.16 kV /480 V/LConn3
  Three-Phase Breaker3/LConn2 -- 672/LConn2 -- PV2 dynamic Load/RConn2 -- PV_Geno_GFL_VSC_at_672/RConn2
  632/LConn1 -- Dyn_Equivalent of Extended Grid 4.160 kV/RConn1
  632/LConn2 -- Dyn_Equivalent of Extended Grid 4.160 kV/RConn2
  632/LConn3 -- Dyn_Equivalent of Extended Grid 4.160 kV/RConn3
  " 672 Yg PQ "/LConn1 -- Three-Phase Breaker3/RConn1
  " 672 Yg PQ "/LConn3 -- Three-Phase Breaker3/RConn3
  " 672 Yg PQ "/LConn2 -- Three-Phase Breaker3/RConn2
  Three-Phase Breaker4/LConn3 -- PV1 dynamic Load/RConn3 -- PV_Geno_GFL_VSC_at_634/RConn3 -- 634/LConn3
  Three-Phase Breaker4/LConn2 -- PV1 dynamic Load/RConn2 -- PV_Geno_GFL_VSC_at_634/RConn2 -- 634/LConn2
  " 634 Yg PQ 1"/LConn2 -- Three-Phase Breaker4/RConn2
  XFM-634 4.16 kV /480 V/RConn1 -- 634/RConn1
  XFM-634 4.16 kV /480 V/RConn3 -- 634/RConn3
  " 634 Yg PQ 1"/LConn1 -- Three-Phase Breaker4/RConn1
  XFM-634 4.16 kV /480 V/RConn2 -- 634/RConn2
  Three-Phase Breaker3/LConn1 -- 672/LConn1 -- PV2 dynamic Load/RConn1 -- PV_Geno_GFL_VSC_at_672/RConn1
  672/RConn1 -- XFM-671 4.16 kV /480 V/RConn1
  672/RConn2 -- XFM-671 4.16 kV /480 V/RConn2
  672/RConn3 -- XFM-671 4.16 kV /480 V/RConn3
  PV_Geno_GFL_VSC_at_672/RConn3 -- PV2 dynamic Load/RConn3 -- Three-Phase Breaker3/LConn3 -- 672/LConn3
  Three-Phase Breaker4/LConn1 -- PV_Geno_GFL_VSC_at_634/RConn1 -- PV1 dynamic Load/RConn1 -- 634/LConn1
  Series RLC Branch3/RConn1 -- 645/RConn1
  646/RConn2 -- " 646 Yg PQ"/LConn2
  646/RConn3 -- " 646 Yg PQ"/LConn3
  Series RLC Branch4/LConn1 -- 684/LConn2
  652-684b/LConn1 -- 684/RConn2 -- 611-684b/RConn1
  652-684b/RConn1 -- 652/LConn2
  652-684c/RConn1 -- 652/LConn3
  611-684b/LConn1 -- 611/LConn2
  611-684/LConn1 -- 611/LConn1
  611/RConn2 -- 611 Yg L/LConn2 -- 611 Yg Z/LConn2
  611/RConn1 -- 611 Yg L/LConn1 -- 611 Yg Z/LConn1
  Three-Phase Breaker4/RConn3 -- " 634 Yg PQ 1"/LConn3
  652/RConn1 -- " 652 Yg Z"/LConn1
  " 652 Yg Z"/LConn2 -- 652/RConn2
  " 652 Yg Z"/LConn3 -- 652/RConn3
  671-680/RConn1 -- XFM-680 4.16 kV /480 V/LConn1
  671-2/RConn1 -- XFM-680 4.16 kV /480 V/LConn2
  671-3/RConn1 -- XFM-680 4.16 kV /480 V/LConn3
  XFM-680 4.16 kV /480 V/RConn1 -- 680/RConn1
  XFM-680 4.16 kV /480 V/RConn2 -- 680/RConn2
  XFM-680 4.16 kV /480 V/RConn3 -- 680/RConn3
  680/LConn1 -- PV1 dynamic Load3/RConn1 -- PV_Geno_GFL_VSC_at_680/RConn1 -- Three-Phase Breaker1/LConn1
  680/LConn2 -- PV1 dynamic Load3/RConn2 -- PV_Geno_GFL_VSC_at_680/RConn2 -- Three-Phase Breaker1/LConn2
  680/LConn3 -- PV1 dynamic Load3/RConn3 -- PV_Geno_GFL_VSC_at_680/RConn3 -- Three-Phase Breaker1/LConn3
  Three-Phase Breaker1/RConn1 -- " 680 Yg PQ "/LConn1
  Three-Phase Breaker1/RConn2 -- " 680 Yg PQ "/LConn2
  Three-Phase Breaker1/RConn3 -- " 680 Yg PQ "/LConn3

== system power_13NodeTestFeeder_4VSC_PV_DEG_symmtrc_loads_/Dyn_Equivalent of Extended Grid 4.160 kV ==
  fg : Inport
  Clock : Clock
  Constant1 : Constant  Value=U_rms
  Equivalent GDE impedance : spsThreePhaseSeriesRLCBranchLib/Three-Phase Series RLC Branch  LConnTagsString=A|B|C  RConnTagsString=A|B|C  BranchType=RL  Resistance=Rg  Inductance=Lg  Capacitance=1e-6  Measurements=None
  Three-phase system : MATLAB Function  TreatAsAtomicUnit=on
  u-controlled Voltage Source : Subsystem
  a : PMIOPort  Side=Right
  b : PMIOPort  Port=2  Side=Right
  c : PMIOPort  Port=3  Side=Right
  wires:
  Three-phase system/1(v) -> u-controlled Voltage Source/1(u)
  fg/1 -> Three-phase system/1(fg)
  Constant1/1 -> Three-phase system/2(U_rms)
  Clock/1 -> Three-phase system/3(t)
  connections:
  u-controlled Voltage Source/RConn1 -- Equivalent GDE impedance/LConn1
  u-controlled Voltage Source/RConn2 -- Equivalent GDE impedance/LConn2
  u-controlled Voltage Source/RConn3 -- Equivalent GDE impedance/LConn3
  Equivalent GDE impedance/RConn1 -- a/RConn1
  Equivalent GDE impedance/RConn2 -- b/RConn1
  Equivalent GDE impedance/RConn3 -- c/RConn1

== system power_13NodeTestFeeder_4VSC_PV_DEG_symmtrc_loads_/Frequency Dynamics ==
  Ppv : Inport
  Pgrid : Inport  Port=2
  dPreq : Inport  Port=3
  Add : Sum
  Constant : Constant  Value=fg
  Divide : Product  Inputs=*/
  Gain : Gain  Gain=fg^2/(2*Sn*H)
  Gain1 : Gain  Gain=Kdroop
  Integrator : Integrator  InitialCondition=60
  Minus : Sum  Inputs=+-
  Saturation : Saturate  UpperLimit=80  LowerLimit=40
  Sum : Sum  Inputs=+--
  fg : Outport
  delta_f : Outport  Port=2
  wires:
  Ppv/1 -> Sum/1
  Pgrid/1 -> Sum/2
  Constant/1 -> Minus/2
  Integrator/1 -> Saturation/1, fg/1  "fg"
  Sum/1 -> Add/2
  Add/1 -> Gain/1
  dPreq/1 -> Add/1
  Divide/1 -> Integrator/1
  Gain/1 -> Divide/1
  Saturation/1 -> Minus/1, Divide/2
  Minus/1 -> Gain1/1, delta_f/1
  Gain1/1 -> Sum/3  "PD"

== system power_13NodeTestFeeder_4VSC_PV_DEG_symmtrc_loads_/Frequency Dynamics linearized (Droop) ==
  dPreq : Inport
  Ppv : Inport  Port=2
  Pgrid : Inport  Port=3
  Constant : Constant  Value=fg
  Gain2 : Gain  Gain=fg/(2*H*Sn)
  Gain3 : Gain  Gain=-fg*Kdroop/(2*H*Sn)
  Integrator : Integrator  InitialCondition=60
  Minus : Sum  Inputs=+-
  Minus1 : Sum  Inputs=++-
  Saturation : Saturate  UpperLimit=80  LowerLimit=40
  Sum : Sum  Inputs=|++
  fg : Outport
  delta_f : Outport  Port=2
  wires:
  Constant/1 -> Minus/2
  Minus/1 -> Gain3/1, delta_f/1
  Integrator/1 -> fg/1, Saturation/1  "fg"
  Sum/1 -> Integrator/1
  Saturation/1 -> Minus/1
  Minus1/1 -> Gain2/1
  Gain2/1 -> Sum/1
  Gain3/1 -> Sum/2
  dPreq/1 -> Minus1/1
  Ppv/1 -> Minus1/2
  Pgrid/1 -> Minus1/3

== system power_13NodeTestFeeder_4VSC_PV_DEG_symmtrc_loads_/Frequency Dynamics linearized (no Droop) ==
  dPreq : Inport
  Ppv : Inport  Port=2
  Pgrid : Inport  Port=3
  Constant : Constant  Value=fg
  Gain2 : Gain  Gain=fg/(2*H*Sn)
  Integrator : Integrator  InitialCondition=60
  Minus : Sum  Inputs=+-
  Minus1 : Sum  Inputs=++-
  Saturation : Saturate  UpperLimit=80  LowerLimit=40
  fg : Outport
  delta_f : Outport  Port=2
  wires:
  Integrator/1 -> Saturation/1, fg/1  "fg"
  Gain2/1 -> Integrator/1
  Minus1/1 -> Gain2/1
  dPreq/1 -> Minus1/1
  Constant/1 -> Minus/2
  Saturation/1 -> Minus/1
  Minus/1 -> delta_f/1
  Ppv/1 -> Minus1/2
  Pgrid/1 -> Minus1/3

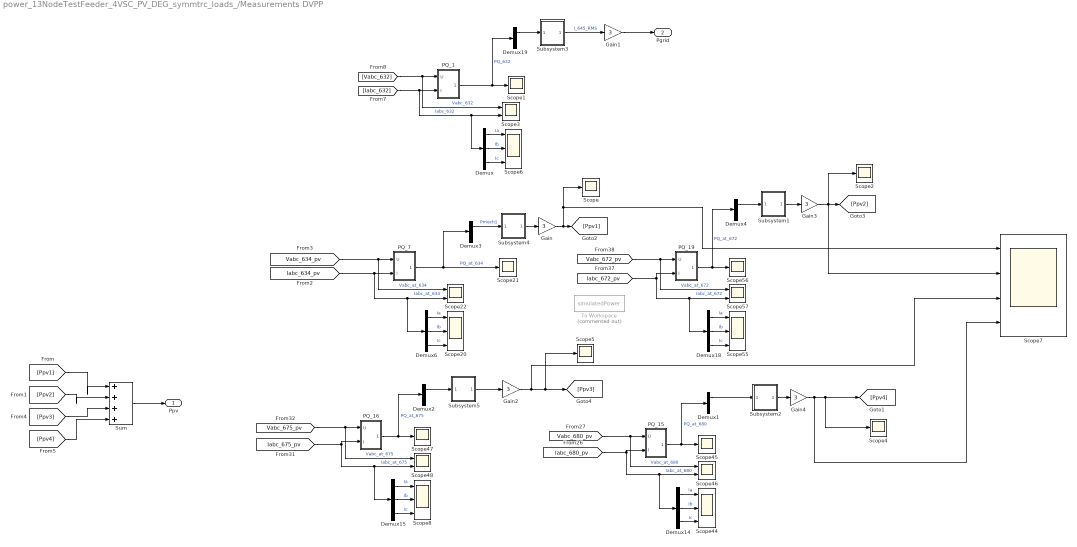
== system power_13NodeTestFeeder_4VSC_PV_DEG_symmtrc_loads_/Measurements DVPP ==
  Demux{,6,14..15,18} (5 alike) : Demux  Outputs=3
  Demux{1..4,19} (5 alike) : Demux  Outputs=2
  Gain{,1..4} (5 alike) : Gain  Gain=3
  PQ_1 : Subsystem
  PQ_15 : Subsystem
  PQ_16 : Subsystem
  PQ_19 : Subsystem
  PQ_7 : Subsystem
  Scope{,1..2,4..5,21,45,47,56} (9 alike) : Scope
  Scope{6,8,20,44,55} (5 alike) : Scope  NumInputPorts=3
  Scope{3,22,46,48,57} (5 alike) : Scope  NumInputPorts=2
  Scope7 : Scope  NumInputPorts=4
  Subsystem1 : Subsystem  mask{fg=fg, Vrms0=0}
      mask prompts: fg "Frequency"; Vrms0 "Initial value"
      mask Display: disp('RMS')
  Subsystem2 : Subsystem  mask{fg=fg, Vrms0=0}
      mask prompts: fg "Frequency"; Vrms0 "Initial value"
      mask Display: disp('RMS')
  Subsystem3 : Subsystem  mask{fg=fg, Vrms0=0}
      mask prompts: fg "Frequency"; Vrms0 "Initial value"
      mask Display: disp('RMS')
  Subsystem4 : Subsystem  mask{fg=fg, Vrms0=0}
      mask prompts: fg "Frequency"; Vrms0 "Initial value"
      mask Display: disp('RMS')
  Subsystem5 : Subsystem  mask{fg=fg, Vrms0=20}
      mask prompts: fg "Frequency"; Vrms0 "Initial value"
      mask Display: disp('RMS')
  Sum : Sum  Inputs=|++++
  To Workspace : ToWorkspace  Commented=on  VariableName=simulatedPower  SaveFormat=Timeseries  SampleTime=Ts
  Ppv : Outport
  Pgrid : Outport  Port=2
  wires:
  Demux19/1 -> Subsystem3/1(In1)
  [Iabc_632] -> Demux/1, Scope3/2, PQ_1/2(I)  "Iabc_632"
  Subsystem3/1(Out1) -> Gain1/1  "I_645_RMS"
  Demux/2 -> Scope6/2  "Ib"
  Demux/1 -> Scope6/1  "Ia"
  [Vabc_632] -> Scope3/1, PQ_1/1(U)  "Vabc_632"
  PQ_1/1(PQ) -> Demux19/1, Scope1/1  "PQ_632"
  Demux/3 -> Scope6/3  "Ic"
  Demux6/2 -> Scope20/2  "Ib"
  Gain4/1 -> Scope7/4, Scope4/1, [Ppv4]
  Gain3/1 -> Scope7/2, Scope2/1, [Ppv2]
  Gain2/1 -> Scope7/3, Scope5/1, [Ppv3]
  Demux14/3 -> Scope44/3  "Ic"
  Gain/1 -> Scope/1, Scope7/1, [Ppv1]
  Subsystem5/1(Out1) -> Gain2/1
  Subsystem2/1(Out1) -> Gain4/1
  Demux6/3 -> Scope20/3  "Ic"
  Demux15/2 -> Scope8/2  "Ib"
  [Ppv1] -> Sum/1
  PQ_7/1(PQ) -> Demux3/1, Scope21/1  "PQ_at_634"
  [Ppv2] -> Sum/2
  Subsystem4/1(Out1) -> Gain/1
  Demux18/1 -> Scope55/1  "Ia"
  [Iabc_680_pv] -> PQ_15/2(I), Scope46/2, Demux14/1  "Iabc_at_680"
  PQ_19/1(PQ) -> Demux4/1, Scope56/1  "PQ_at_672"
  Demux15/1 -> Scope8/1  "Ia"
  Demux14/1 -> Scope44/1  "Ia"
  [Ppv3] -> Sum/3
  Demux4/1 -> Subsystem1/1(In1)
  Demux2/1 -> Subsystem5/1(In1)
  [Vabc_672_pv] -> Scope57/1, PQ_19/1(U)  "Vabc_at_672"
  [Iabc_672_pv] -> PQ_19/2(I), Scope57/2, Demux18/1  "Iabc_at_672"
  Demux18/2 -> Scope55/2  "Ib"
  [Ppv4] -> Sum/4
  Demux6/1 -> Scope20/1  "Ia"
  [Iabc_675_pv] -> PQ_16/2(I), Scope48/2, Demux15/1  "Iabc_at_675"
  Demux1/1 -> Subsystem2/1(In1)
  [Vabc_680_pv] -> Scope46/1, PQ_15/1(U)  "Vabc_at_680"
  [Vabc_634_pv] -> Scope22/1, PQ_7/1(U)  "Vabc_at_634"
  Demux14/2 -> Scope44/2  "Ib"
  [Iabc_634_pv] -> Scope22/2, Demux6/1, PQ_7/2(I)  "Iabc_at_634"
  Demux18/3 -> Scope55/3  "Ic"
  Demux3/1 -> Subsystem4/1(In1)  "Pmech1"
  PQ_16/1(PQ) -> Demux2/1, Scope47/1  "PQ_at_675"
  Subsystem1/1(Out1) -> Gain3/1
  PQ_15/1(PQ) -> Demux1/1, Scope45/1  "PQ_at_680"
  Demux15/3 -> Scope8/3  "Ic"
  [Vabc_675_pv] -> Scope48/1, PQ_16/1(U)  "Vabc_at_675"
  Gain1/1 -> Pgrid/1
  Sum/1 -> Ppv/1

== system power_13NodeTestFeeder_4VSC_PV_DEG_symmtrc_loads_/PV1 dynamic Load ==
  delta_p : Inport
  Bus Selector : BusSelector  OutputSignals=Active power P (W)
  Constant : Constant  Value=ppv_nom
  Gain : Gain  Gain=[-1 0]
  PVG_at_634 : spsThreePhaseVIMeasurementLib/Three-Phase V-I Measurement  VoltageMeasurement=phase-to-ground  SetLabelV=off  LabelV=Vabc_634_pv  Vpu=off  VpuLL=off  CurrentMeasurement=yes  SetLabelI=off  LabelI=Iabc_634_pv  Ipu=off  Pbase=100e6  Vbase=4160  OutputType=Complex  PhasorSimulation=off  PSBequivalent=0
  Scope3 : Scope
  Sum : Sum  Inputs=|++
  Three-Phase Dynamic Load : spsThreePhaseDynamicLoadLib/Three-Phase Dynamic Load  NominalVoltage=[ para_grid.n634YgPQ.V_LN_rms(1)*sqrt(3) 60 ]  ActiveReactivePowers=[ppv_nom 0]  PositiveSequence=[1 0]  ExternalControl=on  NpNq=[1.3 2]  TimeConstants="[0  0  0  0]"  MinimumVoltage=0.7  Tfilter=1e-4  LoadFlowParameters=[4,0,0,0,0]
      settings: LibrarySourceBlock=|
      | sps_lib/Passives/Three-Phase
      | Dynamic Load
  a : PMIOPort  Side=Right
  b : PMIOPort  Port=2  Side=Right
  c : PMIOPort  Port=3  Side=Right
  tag scope: Iabc_634_pv=global, Vabc_634_pv=global
  wires:
  PVG_at_634/1 -> [Vabc_634_pv]
  Bus Selector/1 -> Scope3/1  "<Active power P (W)>"
  PVG_at_634/2 -> [Iabc_634_pv]
  Three-Phase Dynamic Load/1 -> Bus Selector/1
  Gain/1 -> Three-Phase Dynamic Load/1
  delta_p/1 -> Sum/1
  Sum/1 -> Gain/1
  Constant/1 -> Sum/2
  connections:
  PVG_at_634/LConn3 -- Three-Phase Dynamic Load/LConn3
  b/RConn1 -- PVG_at_634/RConn2
  a/RConn1 -- PVG_at_634/RConn1
  PVG_at_634/LConn2 -- Three-Phase Dynamic Load/LConn2
  c/RConn1 -- PVG_at_634/RConn3
  PVG_at_634/LConn1 -- Three-Phase Dynamic Load/LConn1
